simulink model "Sensors"  (Simulink 8.8)
settings: Solver=ode45  StartTime=0.0  StopTime=10.0  RelTol=1e-3  EnableMultiTasking=on
undefined symbols (not defined in the file): Amc_flgAirMassFlowOverride, Amc_uSensMaxValid, Amc_uSensMinValid, Bvc_rVoltDivHigh, Bvc_rVoltDivLow, Bvc_uBattMax, Bvc_uBattMin, Cpc_flgPChargeOverride, Ctc_rPullUp_C, Ctc_uSensMaxValid, Ctc_uSensMinValid, Ctc_uSupply, Egc_facEgasMan, Egc_flgEgasOverride, Egc_stEgasFilt, Egc_tiTEgasFilt, Egc_uSensMaxValid, Egc_uSensMinValid, Mpc_uSensMaxValid, Mpc_uSensMinValid, Mtc_rPullUp_C, Mtc_uSensMaxValid, Mtc_uSensMinValid, Mtc_uSupply, Opc_rpmEngMinOilPressure
libraries: simulink x8
(part 1 of 2)
settings Model: Creator=YAL9FE  LastModifiedBy=ADM4KOR
settings OptimizationCC: ExpressionDepthLimit=2147483647
settings DebuggingCC: SolverPrmCheckMsg=warning
settings ConfigComp: CovSFcnEnable=off

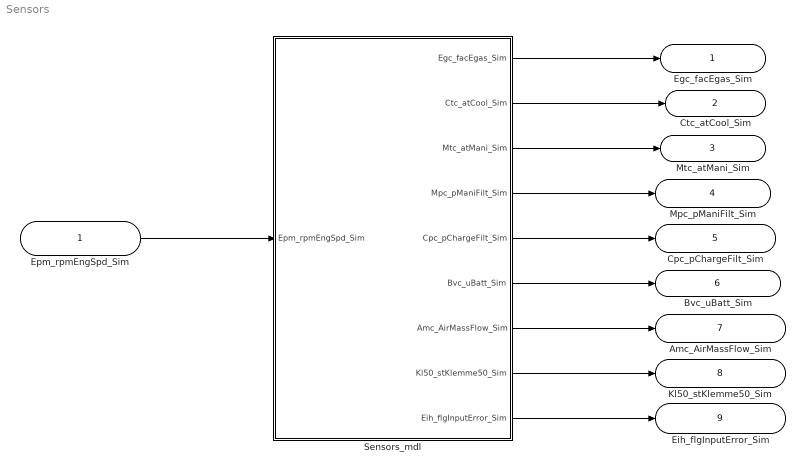
== system Sensors ==
  Epm_rpmEngSpd_Sim : Inport
  Sensors_mdl : Subsystem
  Egc_facEgas_Sim : Outport
  Ctc_atCool_Sim : Outport  Port=2
  Mtc_atMani_Sim : Outport  Port=3
  Mpc_pManiFilt_Sim : Outport  Port=4
  Cpc_pChargeFilt_Sim : Outport  Port=5
  Bvc_uBatt_Sim : Outport  Port=6
  Amc_AirMassFlow_Sim : Outport  Port=7
  Kl50_stKlemme50_Sim : Outport  Port=8
  Eih_flgInputError_Sim : Outport  Port=9
  wires:
  Epm_rpmEngSpd_Sim/1 -> Sensors_mdl/1(Epm_rpmEngSpd_Sim)
  Sensors_mdl/1(Egc_facEgas_Sim) -> Egc_facEgas_Sim/1
  Sensors_mdl/2(Ctc_atCool_Sim) -> Ctc_atCool_Sim/1
  Sensors_mdl/3(Mtc_atMani_Sim) -> Mtc_atMani_Sim/1
  Sensors_mdl/4(Mpc_pManiFilt_Sim) -> Mpc_pManiFilt_Sim/1
  Sensors_mdl/5(Cpc_pChargeFilt_Sim) -> Cpc_pChargeFilt_Sim/1
  Sensors_mdl/6(Bvc_uBatt_Sim) -> Bvc_uBatt_Sim/1
  Sensors_mdl/7(Amc_AirMassFlow_Sim) -> Amc_AirMassFlow_Sim/1
  Sensors_mdl/8(Kl50_stKlemme50_Sim) -> Kl50_stKlemme50_Sim/1
  Sensors_mdl/9(Eih_flgInputError_Sim) -> Eih_flgInputError_Sim/1

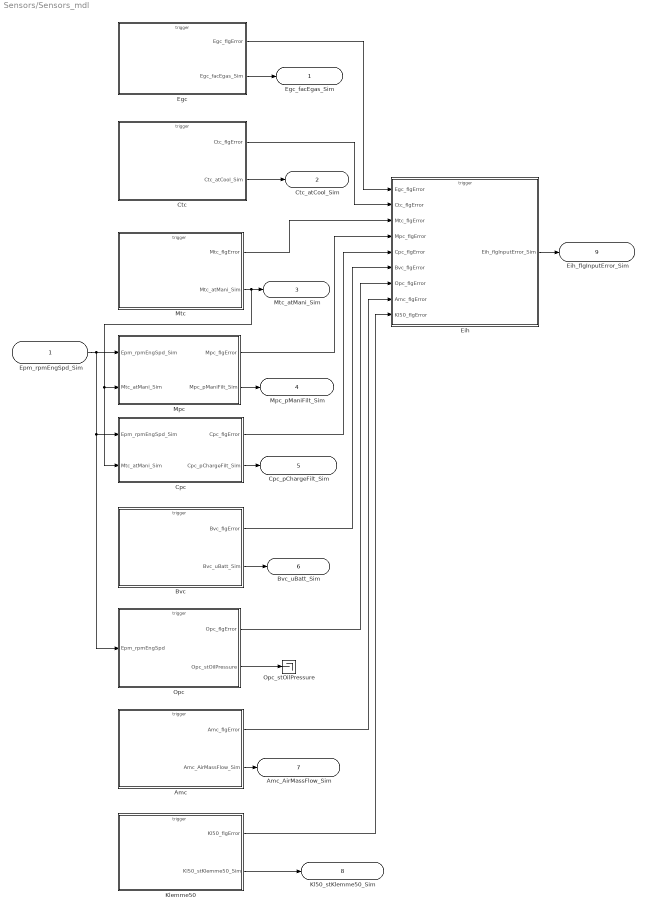
== system Sensors/Sensors_mdl ==
  Epm_rpmEngSpd_Sim : Inport
  Amc : Subsystem  mask(Sensors){}
      mask help: AirMassFlowMeter
      mask Display:
      | image(imread('AirMassFlowMeter.jpg'))
      | port_label('output',1,'Amc_flgError')
      | port_label('output',2,'Amc_AirMassFlow_Sim')
  Bvc : Subsystem  mask(Sensors){}
      mask help: BatteryVoltage
      mask Display:
      | image(imread('BatteryVoltage.jpg'))
      | port_label('output',1,'Bvc_flgError')
      | port_label('output',2,'Bvc_uBatt_Sim')
  Cpc : Subsystem  mask(Sensors){}
      mask help: ChargingPressure
      mask Display:
      | image(imread('ChargingPressure.jpg'))
      | port_label('input',1,'Epm_rpmEngSpd_Sim')
      | port_label('input',2,'Mtc_atMani_Sim')
      | port_label('output',1,'Cpc_flgError')
      | port_label('output',2,'Cpc_pChargeFilt_Sim')
  Ctc : Subsystem  mask(Sensors){}
      mask help: CoolantTemperature
      mask Display:
      | image(imread('CoolantTemperature.jpg'))
      | port_label('output',1,'Ctc_flgError')
      | port_label('output',2,'Ctc_atCool_Sim')
  Egc : Subsystem  mask(Sensors){}
      mask help: Egas
      mask Display:
      | image(imread('Egas.jpg'))
      | port_label('output',1,'Egc_flgError')
      | port_label('output',2,'Egc_facEgas_Sim')
  Eih : Subsystem  mask(Functions){}
      mask help: ErrorInput
      mask Display:
      | image(imread('ErrorInput.jpg'))
      | port_label('input',1,'Egc_flgError')
      | port_label('input',2,'Ctc_flgError')
      | port_label('input',3,'Mtc_flgError')
      | port_label('input',4,'Mpc_flgError')
      | port_label('input',5,'Cpc_flgError')
      | port_label('input',6,'Bvc_flgError')
      | port_label('input',7,'Opc_flgError')
      | port_label('input',8,'Amc_flgError')
      | port_label('input',9,'Kl50_flgError')
      | port_label('output',1,'Eih_flgInputError_Sim')
  Klemme50 : Subsystem  mask(Sensors){}
      mask help: Klemme50
      mask Display:
      | image(imread('Klemme50.jpg'))
      | port_label('output',1,'Kl50_flgError')
      | port_label('output',2,'Kl50_stKlemme50_Sim')
  Mpc : Subsystem  mask(Sensors){}
      mask help: ManifoldPressure
      mask Display:
      | image(imread('ManifoldPressure.jpg'))
      | port_label('input',1,'Epm_rpmEngSpd_Sim')
      | port_label('input',2,'Mtc_atMani_Sim')
      | port_label('output',1,'Mpc_flgError')
      | port_label('output',2,'Mpc_pManiFilt_Sim')
  Mtc : Subsystem  mask(Sensors){}
      mask help: ManifoldTemperature
      mask Display:
      | image(imread('ManifoldTemperature.jpg'))
      | port_label('output',1,'Mtc_flgError')
      | port_label('output',2,'Mtc_atMani_Sim')
  Opc : Subsystem  mask(Sensors){}
      mask help: OilPressure
      mask Display:
      | image(imread('OilPressure.jpg'))
      | port_label('input',1,'Epm_rpmEngSpd')
      | port_label('output',1,'Opc_flgError')
      | port_label('output',2,'Opc_stOilPressure')
  Opc_stOilPressure : Terminator
  Egc_facEgas_Sim : Outport
  Ctc_atCool_Sim : Outport  Port=2
  Mtc_atMani_Sim : Outport  Port=3
  Mpc_pManiFilt_Sim : Outport  Port=4
  Cpc_pChargeFilt_Sim : Outport  Port=5
  Bvc_uBatt_Sim : Outport  Port=6
  Amc_AirMassFlow_Sim : Outport  Port=7
  Kl50_stKlemme50_Sim : Outport  Port=8
  Eih_flgInputError_Sim : Outport  Port=9
  wires:
  Eih/1(Eih_flgInputError_Sim) -> Eih_flgInputError_Sim/1
  Egc/2(Egc_facEgas_Sim) -> Egc_facEgas_Sim/1
  Egc/1(Egc_flgError) -> Eih/1(Egc_flgError)
  Cpc/1(Cpc_flgError) -> Eih/5(Cpc_flgError)
  Mpc/2(Mpc_pManiFilt_Sim) -> Mpc_pManiFilt_Sim/1
  Klemme50/2(Kl50_stKlemme50_Sim) -> Kl50_stKlemme50_Sim/1
  Ctc/1(Ctc_flgError) -> Eih/2(Ctc_flgError)
  Ctc/2(Ctc_atCool_Sim) -> Ctc_atCool_Sim/1
  Mtc/1(Mtc_flgError) -> Eih/3(Mtc_flgError)
  Mtc/2(Mtc_atMani_Sim) -> Mtc_atMani_Sim/1, Cpc/2(Mtc_atMani_Sim), Mpc/2(Mtc_atMani_Sim)
  Mpc/1(Mpc_flgError) -> Eih/4(Mpc_flgError)
  Klemme50/1(Kl50_flgError) -> Eih/9(Kl50_flgError)
  Amc/2(Amc_AirMassFlow_Sim) -> Amc_AirMassFlow_Sim/1
  Epm_rpmEngSpd_Sim/1 -> Opc/1(Epm_rpmEngSpd), Cpc/1(Epm_rpmEngSpd_Sim), Mpc/1(Epm_rpmEngSpd_Sim)
  Bvc/1(Bvc_flgError) -> Eih/6(Bvc_flgError)
  Bvc/2(Bvc_uBatt_Sim) -> Bvc_uBatt_Sim/1
  Opc/1(Opc_flgError) -> Eih/7(Opc_flgError)
  Opc/2(Opc_stOilPressure) -> Opc_stOilPressure/1
  Cpc/2(Cpc_pChargeFilt_Sim) -> Cpc_pChargeFilt_Sim/1
  Amc/1(Amc_flgError) -> Eih/8(Amc_flgError)

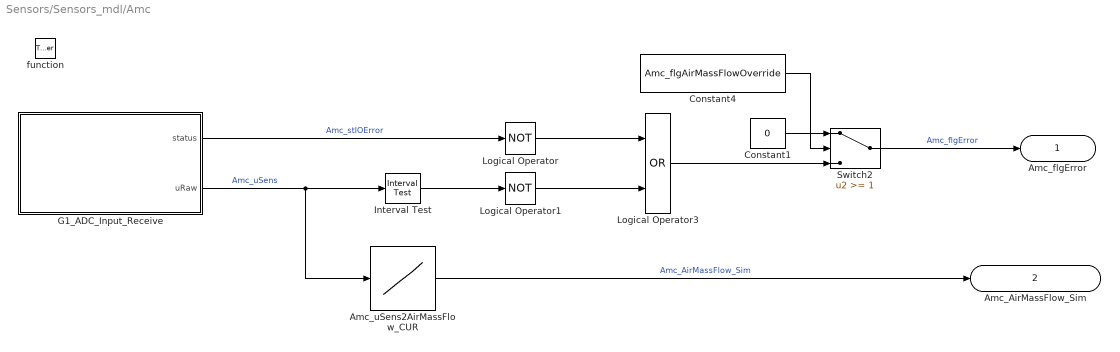
== system Sensors/Sensors_mdl/Amc ==
  function : TriggerPort  TriggerType=function-call  VariantControl=(inherit)
  Amc_uSens2AirMassFlow_CUR : Lookup_n-D  NumberOfTableDimensions=1  BreakpointsForDimension1=[1:3]  BreakpointsForDimension1DataTypeStr=Inherit: Inherit from 'Breakpoint data'  Table=[1 3 7]  TableDataTypeStr=Inherit: Inherit from 'Table data'  ExtrapMethod=Clip  OutDataTypeStr=Inherit: Inherit from 'Table data'  InputSameDT=on
  Constant1 : Constant  Value=0  OutDataTypeStr=boolean
  Constant4 : Constant  Value=Amc_flgAirMassFlowOverride
  G1_ADC_Input_Receive : Subsystem  mask{ChannelName=I_A_AN21}
      mask prompts: ChannelName "Channel name"
      mask init:
      | ehooks_medc17flex_devlib_io_block('mask_init');
      settings: AttributesFormatString=Channel name: '%<ChannelName>'
      mask TypeOptions ChannelName: <empty> | I_A_AN01 | I_A_AN02 | I_A_AN03 | I_A_AN05 | I_A_AN06 | I_A_AN07 | I_A_AN08 | I_A_AN10 | I_A_AN11 | I_A_AN12 | I_A_AN13 | I_A_AN14 | I_A_AN15 | I_A_AN16 | I_A_AN17 | I_A_AN18 | I_A_AN19 | I_A_AN20 | I_A_AN21 | I_A_AN23 | I_A_AN32 | I_A_AN35 | I_A_AN36 | I_A_AN37 | I_A_AN39 | I_A_AN100 | I_A_AN101 | I_A_AN103 | I_A_AN104 | I_A_AN105 | I_A_AN106
      mask Display: image(imread('Input_Analog.jpg'))
  Interval Test : simulink/Logic and Bit Operations/Interval Test  IntervalClosedRight=on  uplimit=Amc_uSensMaxValid  IntervalClosedLeft=on  lowlimit=Amc_uSensMinValid  OutDataTypeStr=boolean
  Logical Operator : Logic  Operator=NOT  AllPortsSameDT=off  OutDataTypeStr=boolean
  Logical Operator1 : Logic  Operator=NOT  AllPortsSameDT=off  OutDataTypeStr=boolean
  Logical Operator3 : Logic  Operator=OR  AllPortsSameDT=off  OutDataTypeStr=boolean
  Switch2 : Switch  Threshold=1
  Amc_flgError : Outport
  Amc_AirMassFlow_Sim : Outport  Port=2
  wires:
  G1_ADC_Input_Receive/1(status) -> Logical Operator/1  "Amc_stIOError"
  G1_ADC_Input_Receive/2(uRaw) -> Amc_uSens2AirMassFlow_CUR/1, Interval Test/1  "Amc_uSens"
  Interval Test/1 -> Logical Operator1/1
  Logical Operator/1 -> Logical Operator3/1
  Logical Operator1/1 -> Logical Operator3/2
  Switch2/1 -> Amc_flgError/1  "Amc_flgError"
  Amc_uSens2AirMassFlow_CUR/1 -> Amc_AirMassFlow_Sim/1  "Amc_AirMassFlow_Sim"
  Constant1/1 -> Switch2/1
  Logical Operator3/1 -> Switch2/3
  Constant4/1 -> Switch2/2

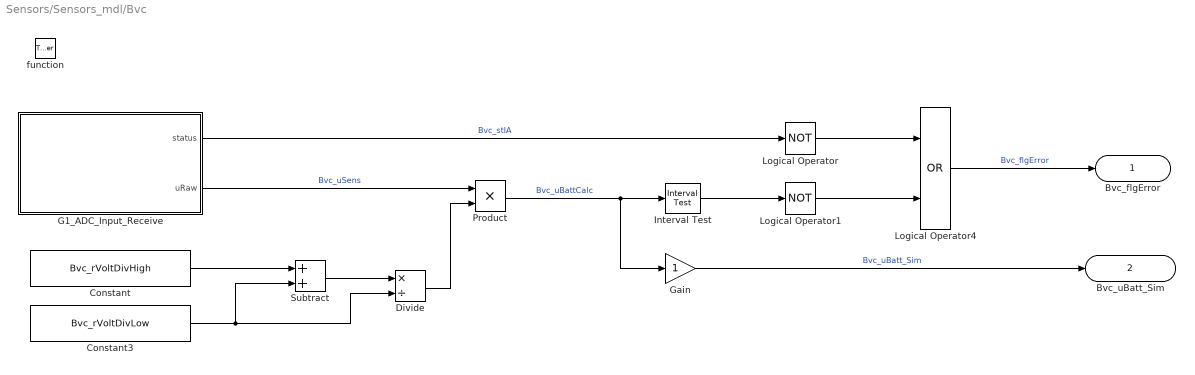
== system Sensors/Sensors_mdl/Bvc ==
  function : TriggerPort  TriggerType=function-call  VariantControl=(inherit)
  Constant : Constant  Value=Bvc_rVoltDivHigh
  Constant3 : Constant  Value=Bvc_rVoltDivLow
  Divide : Product  Inputs=*/  OutDataTypeStr=Inherit: Same as first input
  G1_ADC_Input_Receive : Subsystem  mask{ChannelName=I_A_AN16}
      mask prompts: ChannelName "Channel name"
      mask init:
      | ehooks_medc17flex_devlib_io_block('mask_init');
      settings: AttributesFormatString=Channel name: '%<ChannelName>'
      mask TypeOptions ChannelName: <empty> | I_A_AN01 | I_A_AN02 | I_A_AN03 | I_A_AN05 | I_A_AN06 | I_A_AN07 | I_A_AN08 | I_A_AN10 | I_A_AN11 | I_A_AN12 | I_A_AN13 | I_A_AN14 | I_A_AN15 | I_A_AN16 | I_A_AN17 | I_A_AN18 | I_A_AN19 | I_A_AN20 | I_A_AN21 | I_A_AN23 | I_A_AN32 | I_A_AN35 | I_A_AN36 | I_A_AN37 | I_A_AN39 | I_A_AN100 | I_A_AN101 | I_A_AN103 | I_A_AN104 | I_A_AN105 | I_A_AN106
      mask Display: image(imread('Input_Analog.jpg'))
  Gain : Gain
  Interval Test : simulink/Logic and Bit Operations/Interval Test  IntervalClosedRight=on  uplimit=Bvc_uBattMax  IntervalClosedLeft=on  lowlimit=Bvc_uBattMin  OutDataTypeStr=boolean
  Logical Operator : Logic  Operator=NOT  AllPortsSameDT=off  OutDataTypeStr=boolean
  Logical Operator1 : Logic  Operator=NOT  AllPortsSameDT=off  OutDataTypeStr=boolean
  Logical Operator4 : Logic  Operator=OR  AllPortsSameDT=off  OutDataTypeStr=boolean
  Product : Product  OutDataTypeStr=Inherit: Same as first input
  Subtract : Sum  OutDataTypeStr=Inherit: Same as first input
  Bvc_flgError : Outport
  Bvc_uBatt_Sim : Outport  Port=2
  wires:
  G1_ADC_Input_Receive/1(status) -> Logical Operator/1  "Bvc_stIA"
  Interval Test/1 -> Logical Operator1/1
  Logical Operator/1 -> Logical Operator4/1
  Logical Operator1/1 -> Logical Operator4/2
  Logical Operator4/1 -> Bvc_flgError/1  "Bvc_flgError"
  Constant/1 -> Subtract/1
  Constant3/1 -> Subtract/2, Divide/2
  Subtract/1 -> Divide/1
  Product/1 -> Gain/1, Interval Test/1  "Bvc_uBattCalc"
  G1_ADC_Input_Receive/2(uRaw) -> Product/1  "Bvc_uSens"
  Divide/1 -> Product/2
  Gain/1 -> Bvc_uBatt_Sim/1  "Bvc_uBatt_Sim"

== system Sensors/Sensors_mdl/Cpc ==
  Epm_rpmEngSpd_Sim : Inport
  Mtc_atMani_Sim : Inport  Port=2
  Cpc_calc : Subsystem  mask(Sensors){}
      mask help: ChargingPressureCalc
      mask Display:
      | image(imread('ManifoldPressure.jpg'))
      | port_label('input',1,'Epm_rpmEngSpd')
      | port_label('input',2,'Cpc_pMani')
      | port_label('input',3,'Cpc_flgError')
      | port_label('output',1,'Cpc_pChargeFilt_Sim')
  Cpc_get : Subsystem  mask(Sensors){}
      mask help: ChargingPressureGet
      mask Display:
      | image(imread('ManifoldPressure.jpg'))
      | port_label('input',1,'Mtc_atMani')
      | port_label('output',1,'Cpc_flgError')
      | port_label('output',2,'Cpc_pMani')
  Cpc_flgError : Outport
  Cpc_pChargeFilt_Sim : Outport  Port=2
  wires:
  Cpc_calc/1(Cpc_pChargeFilt_Sim) -> Cpc_pChargeFilt_Sim/1
  Cpc_get/2(Cpc_pMani) -> Cpc_calc/2(Cpc_pMani)
  Epm_rpmEngSpd_Sim/1 -> Cpc_calc/1(Epm_rpmEngSpd_Sim)
  Cpc_get/1(Cpc_flgError) -> Cpc_calc/3(Cpc_flgError), Cpc_flgError/1
  Mtc_atMani_Sim/1 -> Cpc_get/1(Mtc_atMani_Sim)

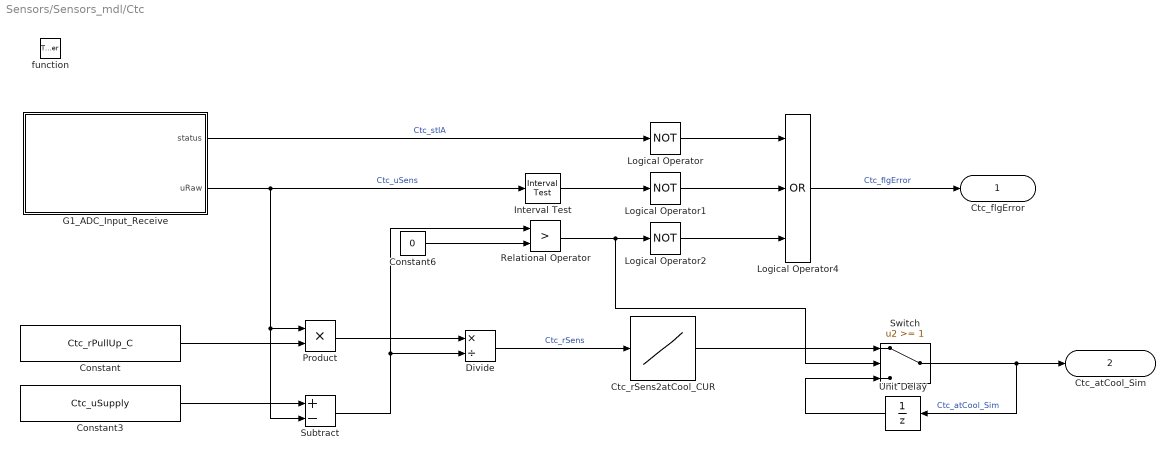
== system Sensors/Sensors_mdl/Ctc ==
  function : TriggerPort  TriggerType=function-call  VariantControl=(inherit)
  Constant : Constant  Value=Ctc_rPullUp_C
  Constant3 : Constant  Value=Ctc_uSupply
  Constant6 : Constant  Value=0  OutDataTypeStr=single
  Ctc_rSens2atCool_CUR : Lookup_n-D  NumberOfTableDimensions=1  BreakpointsForDimension1=[1:3]  BreakpointsForDimension1DataTypeStr=Inherit: Inherit from 'Breakpoint data'  Table=[1 3 4 ]  TableDataTypeStr=Inherit: Inherit from 'Table data'  ExtrapMethod=Clip  OutDataTypeStr=Inherit: Inherit from 'Table data'  InputSameDT=on
  Divide : Product  Inputs=*/  OutDataTypeStr=Inherit: Same as first input
  G1_ADC_Input_Receive : Subsystem  mask{ChannelName=I_A_AN10}
      mask prompts: ChannelName "Channel name"
      mask init:
      | ehooks_medc17flex_devlib_io_block('mask_init');
      settings: AttributesFormatString=Channel name: '%<ChannelName>'
      mask TypeOptions ChannelName: <empty> | I_A_AN01 | I_A_AN02 | I_A_AN03 | I_A_AN05 | I_A_AN06 | I_A_AN07 | I_A_AN08 | I_A_AN10 | I_A_AN11 | I_A_AN12 | I_A_AN13 | I_A_AN14 | I_A_AN15 | I_A_AN16 | I_A_AN17 | I_A_AN18 | I_A_AN19 | I_A_AN20 | I_A_AN21 | I_A_AN23 | I_A_AN32 | I_A_AN35 | I_A_AN36 | I_A_AN37 | I_A_AN39 | I_A_AN100 | I_A_AN101 | I_A_AN103 | I_A_AN104 | I_A_AN105 | I_A_AN106
      mask Display: image(imread('Input_Analog.jpg'))
  Interval Test : simulink/Logic and Bit Operations/Interval Test  IntervalClosedRight=on  uplimit=Ctc_uSensMaxValid  IntervalClosedLeft=on  lowlimit=Ctc_uSensMinValid  OutDataTypeStr=boolean
  Logical Operator : Logic  Operator=NOT  AllPortsSameDT=off  OutDataTypeStr=boolean
  Logical Operator1 : Logic  Operator=NOT  AllPortsSameDT=off  OutDataTypeStr=boolean
  Logical Operator2 : Logic  Operator=NOT  AllPortsSameDT=off  OutDataTypeStr=boolean
  Logical Operator4 : Logic  Operator=OR  Inputs=3  AllPortsSameDT=off  OutDataTypeStr=boolean
  Product : Product  OutDataTypeStr=Inherit: Same as first input
  Relational Operator : RelationalOperator  Operator=>  OutDataTypeStr=boolean  RndMeth=Nearest
  Subtract : Sum  Inputs=+-  OutDataTypeStr=Inherit: Same as first input
  Switch : Switch  Threshold=1
  Unit Delay : UnitDelay  SampleTime=-1
  Ctc_flgError : Outport
  Ctc_atCool_Sim : Outport  Port=2
  wires:
  Logical Operator4/1 -> Ctc_flgError/1  "Ctc_flgError"
  Logical Operator1/1 -> Logical Operator4/2
  Logical Operator/1 -> Logical Operator4/1
  Interval Test/1 -> Logical Operator1/1
  G1_ADC_Input_Receive/2(uRaw) -> Subtract/2, Product/1, Interval Test/1  "Ctc_uSens"
  G1_ADC_Input_Receive/1(status) -> Logical Operator/1  "Ctc_stIA"
  Constant/1 -> Product/2
  Constant3/1 -> Subtract/1
  Product/1 -> Divide/1
  Subtract/1 -> Divide/2, Relational Operator/1
  Constant6/1 -> Relational Operator/2
  Relational Operator/1 -> Logical Operator2/1, Switch/2
  Logical Operator2/1 -> Logical Operator4/3
  Switch/1 -> Ctc_atCool_Sim/1, Unit Delay/1  "Ctc_atCool_Sim"
  Unit Delay/1 -> Switch/3
  Ctc_rSens2atCool_CUR/1 -> Switch/1
  Divide/1 -> Ctc_rSens2atCool_CUR/1  "Ctc_rSens"

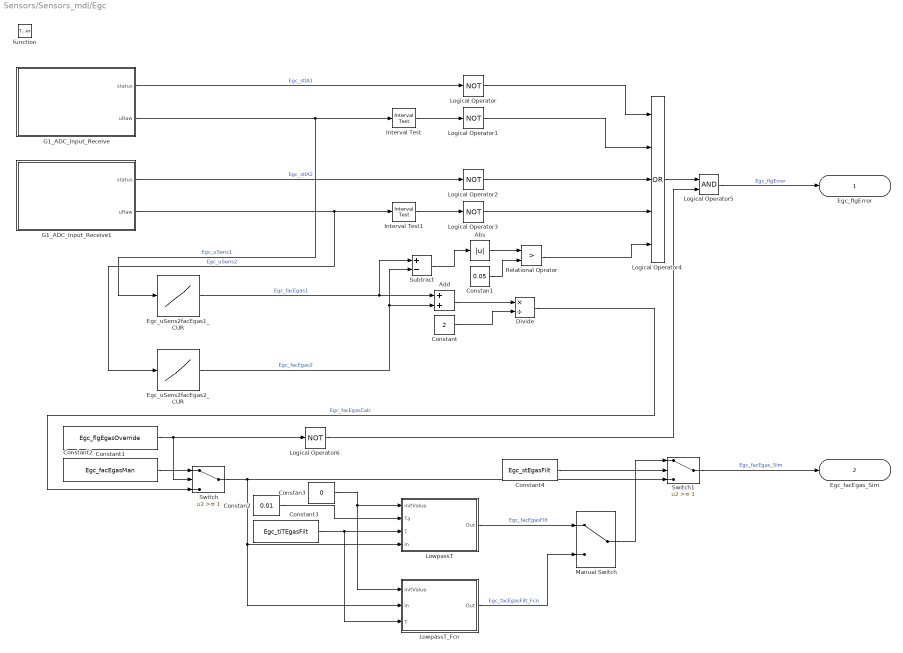
== system Sensors/Sensors_mdl/Egc ==
  function : TriggerPort  TriggerType=function-call  VariantControl=(inherit)
  Abs : Abs
  Add : Sum  OutDataTypeStr=Inherit: Same as first input
  Constan1 : Constant  Value=0.05  OutDataTypeStr=single
  Constan2 : Constant  Value=0.01  OutMin=0  OutDataTypeStr=single
  Constan3 : Constant  Value=0  OutDataTypeStr=single
  Constant : Constant  Value=2  OutDataTypeStr=single
  Constant1 : Constant  Value=Egc_flgEgasOverride
  Constant2 : Constant  Value=Egc_facEgasMan
  Constant3 : Constant  Value=Egc_tiTEgasFilt
  Constant4 : Constant  Value=Egc_stEgasFilt
  Divide : Product  Inputs=*/  OutDataTypeStr=Inherit: Same as first input
  Egc_uSens2facEgas1_CUR : Lookup_n-D  NumberOfTableDimensions=1  BreakpointsForDimension1=[1:3]  BreakpointsForDimension1DataTypeStr=Inherit: Inherit from 'Breakpoint data'  Table=[1 3 9]  TableDataTypeStr=Inherit: Inherit from 'Table data'  ExtrapMethod=Clip  OutDataTypeStr=Inherit: Inherit from 'Table data'  InputSameDT=on
  Egc_uSens2facEgas2_CUR : Lookup_n-D  NumberOfTableDimensions=1  BreakpointsForDimension1=[1:4]  BreakpointsForDimension1DataTypeStr=Inherit: Inherit from 'Breakpoint data'  Table=[1 3 7 9]  TableDataTypeStr=Inherit: Inherit from 'Table data'  ExtrapMethod=Clip  OutDataTypeStr=Inherit: Inherit from 'Table data'  InputSameDT=on
  G1_ADC_Input_Receive : Subsystem  mask{ChannelName=I_A_AN08}
      mask prompts: ChannelName "Channel name"
      mask init:
      | ehooks_medc17flex_devlib_io_block('mask_init');
      settings: AttributesFormatString=Channel name: '%<ChannelName>'
      mask TypeOptions ChannelName: <empty> | I_A_AN01 | I_A_AN02 | I_A_AN03 | I_A_AN05 | I_A_AN06 | I_A_AN07 | I_A_AN08 | I_A_AN10 | I_A_AN11 | I_A_AN12 | I_A_AN13 | I_A_AN14 | I_A_AN15 | I_A_AN16 | I_A_AN17 | I_A_AN18 | I_A_AN19 | I_A_AN20 | I_A_AN21 | I_A_AN23 | I_A_AN32 | I_A_AN35 | I_A_AN36 | I_A_AN37 | I_A_AN39 | I_A_AN100 | I_A_AN101 | I_A_AN103 | I_A_AN104 | I_A_AN105 | I_A_AN106
      mask Display: image(imread('Input_Analog.jpg'))
  G1_ADC_Input_Receive1 : Subsystem  mask{ChannelName=I_A_AN13}
      mask prompts: ChannelName "Channel name"
      mask init:
      | ehooks_medc17flex_devlib_io_block('mask_init');
      settings: AttributesFormatString=Channel name: '%<ChannelName>'
      mask TypeOptions ChannelName: <empty> | I_A_AN01 | I_A_AN02 | I_A_AN03 | I_A_AN05 | I_A_AN06 | I_A_AN07 | I_A_AN08 | I_A_AN10 | I_A_AN11 | I_A_AN12 | I_A_AN13 | I_A_AN14 | I_A_AN15 | I_A_AN16 | I_A_AN17 | I_A_AN18 | I_A_AN19 | I_A_AN20 | I_A_AN21 | I_A_AN23 | I_A_AN32 | I_A_AN35 | I_A_AN36 | I_A_AN37 | I_A_AN39 | I_A_AN100 | I_A_AN101 | I_A_AN103 | I_A_AN104 | I_A_AN105 | I_A_AN106
      mask Display: image(imread('Input_Analog.jpg'))
  Interval Test : simulink/Logic and Bit Operations/Interval Test  IntervalClosedRight=on  uplimit=Egc_uSensMaxValid  IntervalClosedLeft=on  lowlimit=Egc_uSensMinValid  OutDataTypeStr=boolean
  Interval Test1 : simulink/Logic and Bit Operations/Interval Test  IntervalClosedRight=on  uplimit=Egc_uSensMaxValid  IntervalClosedLeft=on  lowlimit=Egc_uSensMinValid  OutDataTypeStr=boolean
  Logical Operator{,1..3,6} (5 alike) : Logic  Operator=NOT  AllPortsSameDT=off  OutDataTypeStr=boolean
  Logical Operator4 : Logic  Operator=OR  Inputs=5  AllPortsSameDT=off  OutDataTypeStr=boolean
  Logical Operator5 : Logic  AllPortsSameDT=off  OutDataTypeStr=boolean
  LowpassT : Subsystem
      mask help: LowpassT
      mask Display: image(imread('LowpassT.jpg'))
  LowpassT_Fcn : Subsystem
      mask help: LowpassT_Fcn
      mask Display: image(imread('LowpassT.jpg'))
  Manual Switch : ManualSwitch
  Relational Oprator : RelationalOperator  Operator=>  OutDataTypeStr=boolean  RndMeth=Nearest
  Subtract : Sum  Inputs=+-  OutDataTypeStr=Inherit: Same as first input
  Switch : Switch  Threshold=1
  Switch1 : Switch  Threshold=1
  Egc_flgError : Outport  InitialOutput=0.0
  Egc_facEgas_Sim : Outport  Port=2  InitialOutput=0.0
  wires:
  Manual Switch/1 -> Switch1/1
  LowpassT/1(Out) -> Manual Switch/1  "Egc_facEgasFilt"
  LowpassT_Fcn/1(Out) -> Manual Switch/2  "Egc_facEgasFilt_Fcn"
  Constant3/1 -> LowpassT_Fcn/3(T), LowpassT/3(T)
  Constan2/1 -> LowpassT/2(Ta)
  Constan3/1 -> LowpassT_Fcn/1(initValue), LowpassT/1(initValue)
  G1_ADC_Input_Receive1/2(uRaw) -> Egc_uSens2facEgas2_CUR/1, Interval Test1/1  "Egc_uSens2"
  G1_ADC_Input_Receive/2(uRaw) -> Egc_uSens2facEgas1_CUR/1, Interval Test/1  "Egc_uSens1"
  Divide/1 -> Switch/3  "Egc_facEgasCalc"
  G1_ADC_Input_Receive/1(status) -> Logical Operator/1  "Egc_stIA1"
  Interval Test/1 -> Logical Operator1/1
  Interval Test1/1 -> Logical Operator3/1
  Logical Operator/1 -> Logical Operator4/1
  Logical Operator1/1 -> Logical Operator4/2
  Logical Operator2/1 -> Logical Operator4/3
  Logical Operator3/1 -> Logical Operator4/4
  Logical Operator4/1 -> Logical Operator5/1
  Logical Operator5/1 -> Egc_flgError/1  "Egc_flgError"
  Egc_uSens2facEgas1_CUR/1 -> Subtract/1, Add/1  "Egc_facEgas1"
  Egc_uSens2facEgas2_CUR/1 -> Subtract/2, Add/2  "Egc_facEgas2"
  Add/1 -> Divide/1
  Constant/1 -> Divide/2
  Subtract/1 -> Abs/1
  Abs/1 -> Relational Oprator/1
  Constan1/1 -> Relational Oprator/2
  Relational Oprator/1 -> Logical Operator4/5
  Constant1/1 -> Logical Operator6/1, Switch/2
  Logical Operator6/1 -> Logical Operator5/2
  Switch/1 -> Switch1/3, LowpassT_Fcn/2(In), LowpassT/4(in)
  Switch1/1 -> Egc_facEgas_Sim/1  "Egc_facEgas_Sim"
  Constant4/1 -> Switch1/2
  G1_ADC_Input_Receive1/1(status) -> Logical Operator2/1  "Egc_stIA2"
  Constant2/1 -> Switch/1

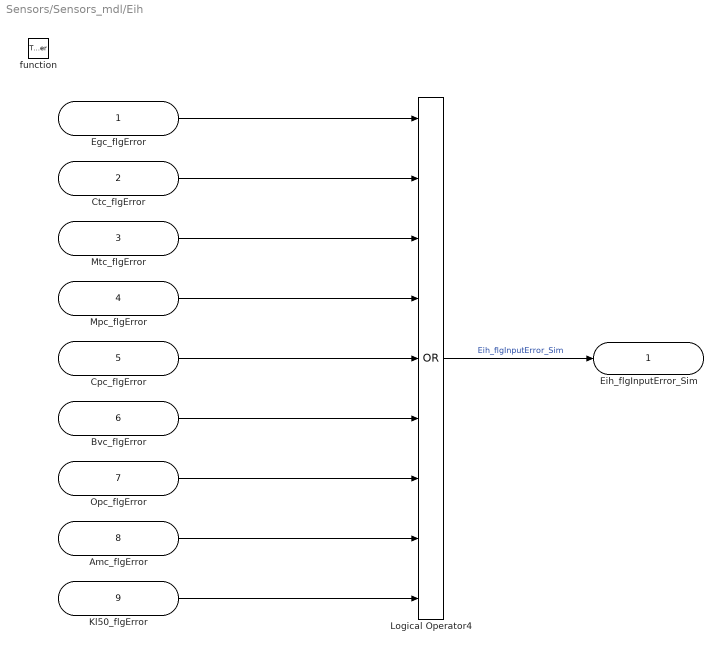
== system Sensors/Sensors_mdl/Eih ==
  Egc_flgError : Inport
  Ctc_flgError : Inport  Port=2
  Mtc_flgError : Inport  Port=3
  Mpc_flgError : Inport  Port=4
  Cpc_flgError : Inport  Port=5
  Bvc_flgError : Inport  Port=6
  Opc_flgError : Inport  Port=7
  Amc_flgError : Inport  Port=8
  Kl50_flgError : Inport  Port=9
  function : TriggerPort  TriggerType=function-call  VariantControl=(inherit)
  Logical Operator4 : Logic  Operator=OR  Inputs=9  AllPortsSameDT=off  OutDataTypeStr=boolean
  Eih_flgInputError_Sim : Outport
  wires:
  Logical Operator4/1 -> Eih_flgInputError_Sim/1  "Eih_flgInputError_Sim"
  Egc_flgError/1 -> Logical Operator4/1
  Ctc_flgError/1 -> Logical Operator4/2
  Mtc_flgError/1 -> Logical Operator4/3
  Mpc_flgError/1 -> Logical Operator4/4
  Cpc_flgError/1 -> Logical Operator4/5
  Bvc_flgError/1 -> Logical Operator4/6
  Opc_flgError/1 -> Logical Operator4/7
  Amc_flgError/1 -> Logical Operator4/8
  Kl50_flgError/1 -> Logical Operator4/9

== system Sensors/Sensors_mdl/Klemme50 ==
  function : TriggerPort  TriggerType=function-call  VariantControl=(inherit)
  G1_Digital_Input_Receive : Subsystem  AncestorBlock=ehooks_medc17flex_G1_lib/Library Blocks/Basic_IO/Inputs/G1_Digital_Input_Receive  mask{ChannelName=I_S_DIG17}
      mask prompts: ChannelName "Channel name"
      mask init:
      | ehooks_medc17flex_devlib_io_block('mask_init');
      settings: AttributesFormatString=Channel name: '%<ChannelName>'
      mask TypeOptions ChannelName: <empty> | I_S_T15 | I_S_DIG02 | I_S_DIG05 | I_S_DIG13 | I_S_DIG14 | I_S_DIG15 | I_S_DIG16 | I_S_DIG17 | I_S_DIG20 | I_S_DIG50
      mask Display: image(imread('Input_Digital.jpg'))
  Logical Operator : Logic  Operator=NOT  AllPortsSameDT=off  OutDataTypeStr=boolean
  Kl50_flgError : Outport
  Kl50_stKlemme50_Sim : Outport  Port=2
  wires:
  Logical Operator/1 -> Kl50_flgError/1  "Kl50_flgError"
  G1_Digital_Input_Receive/1(status) -> Logical Operator/1  "Kl50_stIO"
  G1_Digital_Input_Receive/2(stRaw1) -> Kl50_stKlemme50_Sim/1  "Kl50_stKlemme50_Sim"

== system Sensors/Sensors_mdl/Mpc ==
  Epm_rpmEngSpd_Sim : Inport
  Mtc_atMani_Sim : Inport  Port=2
  Mpc_calc : Subsystem  mask(Sensors){}
      mask help: ManifoldPressureCalc
      mask Display:
      | image(imread('ManifoldPressure.jpg'))
      | port_label('input',1,'Epm_rpmEngSpd')
      | port_label('input',2,'Mpc_pMani')
      | port_label('input',3,'Mpc_flgError')
      | port_label('output',1,'Mpc_pManiFilt')
  Mpc_get : Subsystem  mask(Sensors){}
      mask help: ManifoldPressureGet
      mask Display:
      | image(imread('ManifoldPressure.jpg'))
      | port_label('input',1,'Mtc_atMani_Sim')
      | port_label('output',1,'Mpc_flgError')
      | port_label('output',2,'Mpc_pMani')
  Mpc_flgError : Outport
  Mpc_pManiFilt_Sim : Outport  Port=2
  wires:
  Mtc_atMani_Sim/1 -> Mpc_get/1(Mtc_atMani_Sim)
  Mpc_get/1(Mpc_flgError) -> Mpc_flgError/1, Mpc_calc/3(Mpc_flgError)
  Epm_rpmEngSpd_Sim/1 -> Mpc_calc/1(Epm_rpmEngSpd_Sim)
  Mpc_get/2(Mpc_pMani) -> Mpc_calc/2(Mpc_pMani)
  Mpc_calc/1(Mpc_pManiFilt_Sim) -> Mpc_pManiFilt_Sim/1

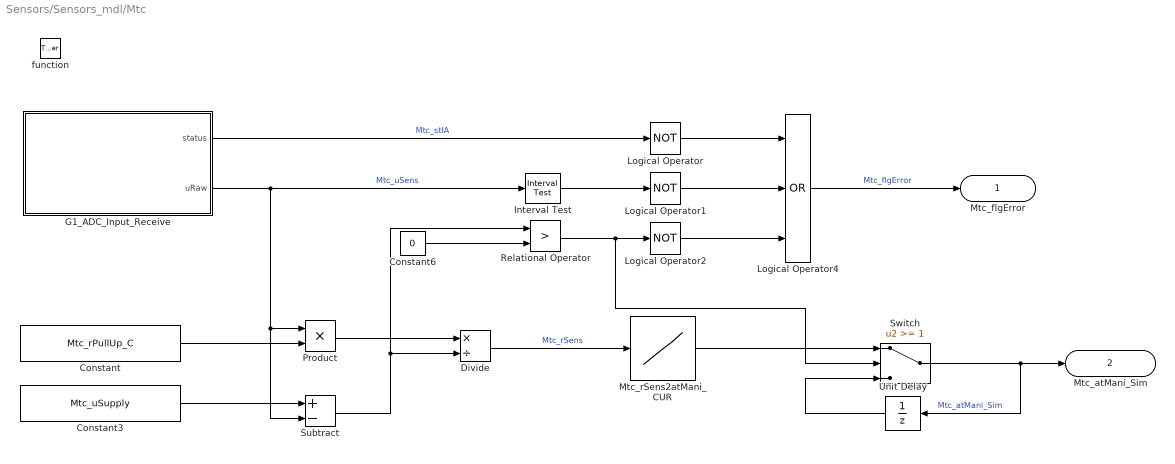
== system Sensors/Sensors_mdl/Mtc ==
  function : TriggerPort  TriggerType=function-call  VariantControl=(inherit)
  Constant : Constant  Value=Mtc_rPullUp_C
  Constant3 : Constant  Value=Mtc_uSupply
  Constant6 : Constant  Value=0  OutDataTypeStr=single
  Divide : Product  Inputs=*/  OutDataTypeStr=single
  G1_ADC_Input_Receive : Subsystem  mask{ChannelName=I_A_AN14}
      mask prompts: ChannelName "Channel name"
      mask init:
      | ehooks_medc17flex_devlib_io_block('mask_init');
      settings: AttributesFormatString=Channel name: '%<ChannelName>'
      mask TypeOptions ChannelName: <empty> | I_A_AN01 | I_A_AN02 | I_A_AN03 | I_A_AN05 | I_A_AN06 | I_A_AN07 | I_A_AN08 | I_A_AN10 | I_A_AN11 | I_A_AN12 | I_A_AN13 | I_A_AN14 | I_A_AN15 | I_A_AN16 | I_A_AN17 | I_A_AN18 | I_A_AN19 | I_A_AN20 | I_A_AN21 | I_A_AN23 | I_A_AN32 | I_A_AN35 | I_A_AN36 | I_A_AN37 | I_A_AN39 | I_A_AN100 | I_A_AN101 | I_A_AN103 | I_A_AN104 | I_A_AN105 | I_A_AN106
      mask Display: image(imread('Input_Analog.jpg'))
  Interval Test : simulink/Logic and Bit Operations/Interval Test  IntervalClosedRight=on  uplimit=Mtc_uSensMaxValid  IntervalClosedLeft=on  lowlimit=Mtc_uSensMinValid  OutDataTypeStr=boolean
  Logical Operator : Logic  Operator=NOT  AllPortsSameDT=off  OutDataTypeStr=boolean
  Logical Operator1 : Logic  Operator=NOT  AllPortsSameDT=off  OutDataTypeStr=boolean
  Logical Operator2 : Logic  Operator=NOT  AllPortsSameDT=off  OutDataTypeStr=boolean
  Logical Operator4 : Logic  Operator=OR  Inputs=3  AllPortsSameDT=off  OutDataTypeStr=boolean
  Mtc_rSens2atMani_CUR : Lookup_n-D  NumberOfTableDimensions=1  BreakpointsForDimension1=[1:3]  BreakpointsForDimension1DataTypeStr=Inherit: Inherit from 'Breakpoint data'  Table=[2 3 6]  TableDataTypeStr=Inherit: Inherit from 'Table data'  ExtrapMethod=Clip  OutDataTypeStr=Inherit: Inherit from 'Table data'  InputSameDT=on
  Product : Product  OutDataTypeStr=Inherit: Same as first input
  Relational Operator : RelationalOperator  Operator=>  OutDataTypeStr=boolean  RndMeth=Nearest
  Subtract : Sum  Inputs=+-  OutDataTypeStr=Inherit: Same as first input
  Switch : Switch  Threshold=1
  Unit Delay : UnitDelay  SampleTime=-1
  Mtc_flgError : Outport
  Mtc_atMani_Sim : Outport  Port=2
  wires:
  Mtc_rSens2atMani_CUR/1 -> Switch/1
  Unit Delay/1 -> Switch/3
  Switch/1 -> Unit Delay/1, Mtc_atMani_Sim/1  "Mtc_atMani_Sim"
  Logical Operator2/1 -> Logical Operator4/3
  Divide/1 -> Mtc_rSens2atMani_CUR/1  "Mtc_rSens"
  Relational Operator/1 -> Switch/2, Logical Operator2/1
  Constant6/1 -> Relational Operator/2
  Subtract/1 -> Relational Operator/1, Divide/2
  Product/1 -> Divide/1
  Constant3/1 -> Subtract/1
  Constant/1 -> Product/2
  G1_ADC_Input_Receive/1(status) -> Logical Operator/1  "Mtc_stIA"
  G1_ADC_Input_Receive/2(uRaw) -> Product/1, Subtract/2, Interval Test/1  "Mtc_uSens"
  Interval Test/1 -> Logical Operator1/1
  Logical Operator/1 -> Logical Operator4/1
  Logical Operator1/1 -> Logical Operator4/2
  Logical Operator4/1 -> Mtc_flgError/1  "Mtc_flgError"

== system Sensors/Sensors_mdl/Opc ==
  Epm_rpmEngSpd : Inport
  function : TriggerPort  TriggerType=function-call  VariantControl=(inherit)
  Constant : Constant  Value=Opc_rpmEngMinOilPressure
  G1_Digital_Input_Receive : Subsystem  AncestorBlock=ehooks_medc17flex_G1_lib/Library Blocks/Basic_IO/Inputs/G1_Digital_Input_Receive  mask{ChannelName=I_S_DIG13}
      mask prompts: ChannelName "Channel name"
      mask init:
      | ehooks_medc17flex_devlib_io_block('mask_init');
      settings: AttributesFormatString=Channel name: '%<ChannelName>'
      mask TypeOptions ChannelName: <empty> | I_S_T15 | I_S_DIG02 | I_S_DIG05 | I_S_DIG13 | I_S_DIG14 | I_S_DIG15 | I_S_DIG16 | I_S_DIG17 | I_S_DIG20 | I_S_DIG50
      mask Display: image(imread('Input_Digital.jpg'))
  Gain : Gain  OutDataTypeStr=Inherit: Same as input
  Logical Operator : Logic  Operator=NOT  AllPortsSameDT=off  OutDataTypeStr=boolean
  Logical Operator1 : Logic  Operator=NOT  AllPortsSameDT=off  OutDataTypeStr=boolean
  Logical Operator3 : Logic  AllPortsSameDT=off  OutDataTypeStr=boolean
  Logical Operator4 : Logic  Operator=OR  AllPortsSameDT=off  OutDataTypeStr=boolean
  Relational Operator : RelationalOperator  Operator=>  OutDataTypeStr=boolean  RndMeth=Nearest
  Opc_flgError : Outport
  Opc_stOilPressure : Outport  Port=2
  wires:
  Gain/1 -> Opc_stOilPressure/1  "Opc_stOilPressure"
  Constant/1 -> Relational Operator/2
  Logical Operator4/1 -> Opc_flgError/1  "Opc_flgError"
  Logical Operator/1 -> Logical Operator4/1
  G1_Digital_Input_Receive/1(status) -> Logical Operator/1  "Opc_stIA"
  Epm_rpmEngSpd/1 -> Relational Operator/1
  Relational Operator/1 -> Logical Operator3/1
  Logical Operator3/1 -> Logical Operator4/2
  Logical Operator1/1 -> Logical Operator3/2
  G1_Digital_Input_Receive/2(stRaw1) -> Logical Operator1/1, Gain/1  "Opc_stSens"

== system Sensors/Sensors_mdl/Amc/G1_ADC_Input_Receive ==
  Data Type Conversion2 : DataTypeConversion  OutMin=0.0  OutMax=5.0  OutDataTypeStr=single
  Data Type Conversion3 : DataTypeConversion  OutMin=0.0  OutMax=1.0  OutDataTypeStr=boolean
  FlexECU_DevLib_FcnAPI_Wrapper_SFcn : S-Function  FunctionName=ehooks_medc17flex_devlib_basic_io_fcncall  Parameters=NoInputPorts, NoOutputPorts, InputPortDataTypes, OutputPortDataTypes, CFunctionArgTypes, CFunctionName, ChannelName  SFunctionDeploymentMode=off  EnableBusSupport=off  mask{NoInputPorts=0, NoOutputPorts=2, InputPortDataTypes=, OutputPortDataTypes=uint8,int16, CFunctionArgTypes=ret,ref, CFunctionName=DevLib_Adc_Get, ChannelName=I_A_AN21}
      mask prompts: NoInputPorts "Number of input ports"; NoOutputPorts "Number of output ports"; InputPortDataTypes "Input port data types"; OutputPortDataTypes "Output port data types"; CFunctionArgTypes "C function argument types"; CFunctionName "C function name"; ChannelName "Channel (pin) name"
      mask Display: disp('EHOOKS FlexECU\nDevLib Wrapper\nS-Function')
  Gain : Gain  Gain=5/1023  OutDataTypeStr=Inherit: Same as input
  status : Outport
  uRaw : Outport  Port=2
  wires:
  Gain/1 -> uRaw/1
  Data Type Conversion2/1 -> Gain/1
  Data Type Conversion3/1 -> status/1
  FlexECU_DevLib_FcnAPI_Wrapper_SFcn/1 -> Data Type Conversion3/1
  FlexECU_DevLib_FcnAPI_Wrapper_SFcn/2 -> Data Type Conversion2/1

== system Sensors/Sensors_mdl/Bvc/G1_ADC_Input_Receive ==
  Data Type Conversion2 : DataTypeConversion  OutMin=0.0  OutMax=5.0  OutDataTypeStr=single
  Data Type Conversion3 : DataTypeConversion  OutMin=0.0  OutMax=1.0  OutDataTypeStr=boolean
  FlexECU_DevLib_FcnAPI_Wrapper_SFcn : S-Function  FunctionName=ehooks_medc17flex_devlib_basic_io_fcncall  Parameters=NoInputPorts, NoOutputPorts, InputPortDataTypes, OutputPortDataTypes, CFunctionArgTypes, CFunctionName, ChannelName  SFunctionDeploymentMode=off  EnableBusSupport=off  mask{NoInputPorts=0, NoOutputPorts=2, InputPortDataTypes=, OutputPortDataTypes=uint8,int16, CFunctionArgTypes=ret,ref, CFunctionName=DevLib_Adc_Get, ChannelName=I_A_AN16}
      mask prompts: NoInputPorts "Number of input ports"; NoOutputPorts "Number of output ports"; InputPortDataTypes "Input port data types"; OutputPortDataTypes "Output port data types"; CFunctionArgTypes "C function argument types"; CFunctionName "C function name"; ChannelName "Channel (pin) name"
      mask Display: disp('EHOOKS FlexECU\nDevLib Wrapper\nS-Function')
  Gain : Gain  Gain=5/1023  OutDataTypeStr=Inherit: Same as input
  status : Outport
  uRaw : Outport  Port=2
  wires:
  Gain/1 -> uRaw/1
  Data Type Conversion2/1 -> Gain/1
  Data Type Conversion3/1 -> status/1
  FlexECU_DevLib_FcnAPI_Wrapper_SFcn/1 -> Data Type Conversion3/1
  FlexECU_DevLib_FcnAPI_Wrapper_SFcn/2 -> Data Type Conversion2/1

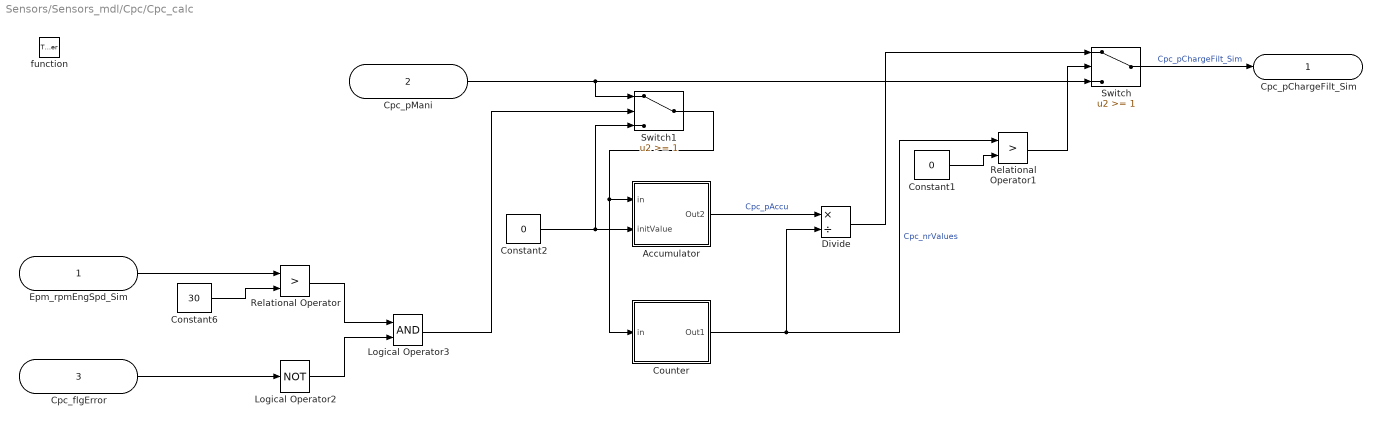
== system Sensors/Sensors_mdl/Cpc/Cpc_calc ==
  Epm_rpmEngSpd_Sim : Inport
  Cpc_pMani : Inport  Port=2
  Cpc_flgError : Inport  Port=3
  function : TriggerPort  TriggerType=function-call  VariantControl=(inherit)
  Accumulator : Subsystem
      mask help: Accumulator
      mask Display: image(imread('Accumulator.jpg'))
  Constant1 : Constant  Value=0  OutDataTypeStr=single
  Constant2 : Constant  Value=0  OutDataTypeStr=single
  Constant6 : Constant  Value=30  OutDataTypeStr=single
  Counter : Subsystem
      mask help: Counter
      mask Display: image(imread('Counter.jpg'))
  Divide : Product  Inputs=*/  OutDataTypeStr=single
  Logical Operator2 : Logic  Operator=NOT  AllPortsSameDT=off  OutDataTypeStr=boolean
  Logical Operator3 : Logic  AllPortsSameDT=off  OutDataTypeStr=boolean
  Relational Operator : RelationalOperator  Operator=>  OutDataTypeStr=boolean  RndMeth=Nearest
  Relational Operator1 : RelationalOperator  Operator=>  OutDataTypeStr=boolean  RndMeth=Nearest
  Switch : Switch  Threshold=1
  Switch1 : Switch  Threshold=1
  Cpc_pChargeFilt_Sim : Outport
  wires:
  Cpc_flgError/1 -> Logical Operator2/1
  Cpc_pMani/1 -> Switch1/1, Switch/3
  Logical Operator2/1 -> Logical Operator3/2
  Relational Operator/1 -> Logical Operator3/1
  Epm_rpmEngSpd_Sim/1 -> Relational Operator/1
  Constant6/1 -> Relational Operator/2
  Counter/1(Out1) -> Divide/2, Relational Operator1/1  "Cpc_nrValues"
  Constant1/1 -> Relational Operator1/2
  Relational Operator1/1 -> Switch/2
  Constant2/1 -> Accumulator/2(initValue), Switch1/3
  Accumulator/1(Out2) -> Divide/1  "Cpc_pAccu"
  Switch/1 -> Cpc_pChargeFilt_Sim/1  "Cpc_pChargeFilt_Sim"
  Divide/1 -> Switch/1
  Logical Operator3/1 -> Switch1/2
  Switch1/1 -> Accumulator/1(in), Counter/1(in)

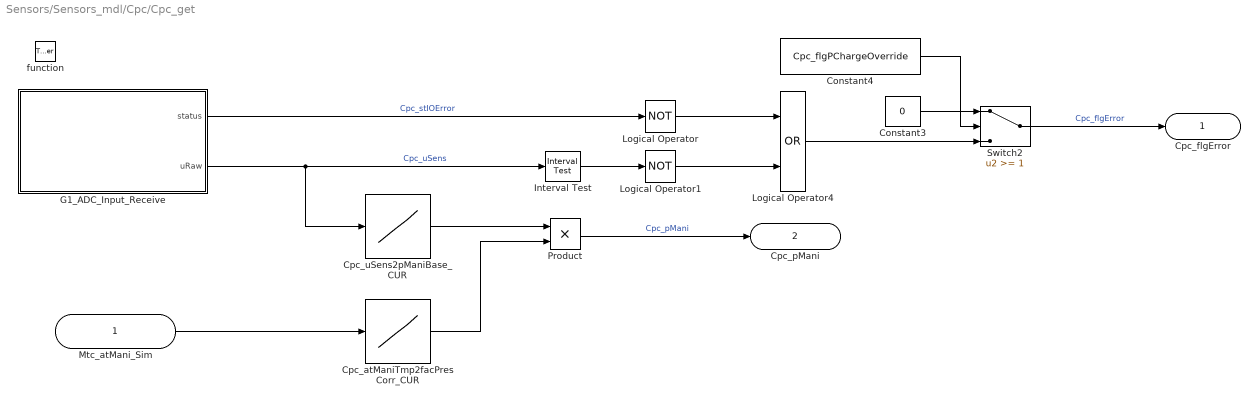
== system Sensors/Sensors_mdl/Cpc/Cpc_get ==
  Mtc_atMani_Sim : Inport
  function : TriggerPort  TriggerType=function-call  VariantControl=(inherit)
  Constant3 : Constant  Value=0  OutDataTypeStr=boolean
  Constant4 : Constant  Value=Cpc_flgPChargeOverride
  Cpc_atManiTmp2facPresCorr_CUR : Lookup_n-D  NumberOfTableDimensions=1  BreakpointsForDimension1=[1:3]  BreakpointsForDimension1DataTypeStr=Inherit: Inherit from 'Breakpoint data'  Table=[6 4 9]  TableDataTypeStr=Inherit: Inherit from 'Table data'  ExtrapMethod=Clip  OutDataTypeStr=Inherit: Inherit from 'Table data'  InputSameDT=on
  Cpc_uSens2pManiBase_CUR : Lookup_n-D  NumberOfTableDimensions=1  BreakpointsForDimension1=[1:3]  BreakpointsForDimension1DataTypeStr=Inherit: Inherit from 'Breakpoint data'  Table=[1 2 5]  TableDataTypeStr=Inherit: Inherit from 'Table data'  ExtrapMethod=Clip  OutDataTypeStr=Inherit: Inherit from 'Table data'  InputSameDT=on
  G1_ADC_Input_Receive : Subsystem  mask{ChannelName=I_A_AN05}
      mask prompts: ChannelName "Channel name"
      mask init:
      | ehooks_medc17flex_devlib_io_block('mask_init');
      settings: AttributesFormatString=Channel name: '%<ChannelName>'
      mask TypeOptions ChannelName: <empty> | I_A_AN01 | I_A_AN02 | I_A_AN03 | I_A_AN05 | I_A_AN06 | I_A_AN07 | I_A_AN08 | I_A_AN10 | I_A_AN11 | I_A_AN12 | I_A_AN13 | I_A_AN14 | I_A_AN15 | I_A_AN16 | I_A_AN17 | I_A_AN18 | I_A_AN19 | I_A_AN20 | I_A_AN21 | I_A_AN23 | I_A_AN32 | I_A_AN35 | I_A_AN36 | I_A_AN37 | I_A_AN39 | I_A_AN100 | I_A_AN101 | I_A_AN103 | I_A_AN104 | I_A_AN105 | I_A_AN106
      mask Display: image(imread('Input_Analog.jpg'))
  Interval Test : simulink/Logic and Bit Operations/Interval Test  IntervalClosedRight=on  uplimit=Mpc_uSensMaxValid  IntervalClosedLeft=on  lowlimit=Mpc_uSensMinValid  OutDataTypeStr=boolean
  Logical Operator : Logic  Operator=NOT  AllPortsSameDT=off  OutDataTypeStr=boolean
  Logical Operator1 : Logic  Operator=NOT  AllPortsSameDT=off  OutDataTypeStr=boolean
  Logical Operator4 : Logic  Operator=OR  AllPortsSameDT=off  OutDataTypeStr=boolean
  Product : Product  OutDataTypeStr=Inherit: Same as first input
  Switch2 : Switch  Threshold=1
  Cpc_flgError : Outport
  Cpc_pMani : Outport  Port=2
  wires:
  Cpc_atManiTmp2facPresCorr_CUR/1 -> Product/2
  Cpc_uSens2pManiBase_CUR/1 -> Product/1
  Mtc_atMani_Sim/1 -> Cpc_atManiTmp2facPresCorr_CUR/1
  Product/1 -> Cpc_pMani/1  "Cpc_pMani"
  G1_ADC_Input_Receive/1(status) -> Logical Operator/1  "Cpc_stIOError"
  G1_ADC_Input_Receive/2(uRaw) -> Cpc_uSens2pManiBase_CUR/1, Interval Test/1  "Cpc_uSens"
  Interval Test/1 -> Logical Operator1/1
  Logical Operator/1 -> Logical Operator4/1
  Logical Operator1/1 -> Logical Operator4/2
  Switch2/1 -> Cpc_flgError/1  "Cpc_flgError"
  Logical Operator4/1 -> Switch2/3
  Constant3/1 -> Switch2/1
  Constant4/1 -> Switch2/2

== system Sensors/Sensors_mdl/Ctc/G1_ADC_Input_Receive ==
  Data Type Conversion2 : DataTypeConversion  OutMin=0.0  OutMax=5.0  OutDataTypeStr=single
  Data Type Conversion3 : DataTypeConversion  OutMin=0.0  OutMax=1.0  OutDataTypeStr=boolean
  FlexECU_DevLib_FcnAPI_Wrapper_SFcn : S-Function  FunctionName=ehooks_medc17flex_devlib_basic_io_fcncall  Parameters=NoInputPorts, NoOutputPorts, InputPortDataTypes, OutputPortDataTypes, CFunctionArgTypes, CFunctionName, ChannelName  SFunctionDeploymentMode=off  EnableBusSupport=off  mask{NoInputPorts=0, NoOutputPorts=2, InputPortDataTypes=, OutputPortDataTypes=uint8,int16, CFunctionArgTypes=ret,ref, CFunctionName=DevLib_Adc_Get, ChannelName=I_A_AN10}
      mask prompts: NoInputPorts "Number of input ports"; NoOutputPorts "Number of output ports"; InputPortDataTypes "Input port data types"; OutputPortDataTypes "Output port data types"; CFunctionArgTypes "C function argument types"; CFunctionName "C function name"; ChannelName "Channel (pin) name"
      mask Display: disp('EHOOKS FlexECU\nDevLib Wrapper\nS-Function')
  Gain : Gain  Gain=5/1023  OutDataTypeStr=Inherit: Same as input
  status : Outport
  uRaw : Outport  Port=2
  wires:
  FlexECU_DevLib_FcnAPI_Wrapper_SFcn/2 -> Data Type Conversion2/1
  FlexECU_DevLib_FcnAPI_Wrapper_SFcn/1 -> Data Type Conversion3/1
  Data Type Conversion3/1 -> status/1
  Data Type Conversion2/1 -> Gain/1
  Gain/1 -> uRaw/1

== system Sensors/Sensors_mdl/Egc/G1_ADC_Input_Receive ==
  Data Type Conversion : DataTypeConversion  OutMin=0.0  OutMax=5.0  OutDataTypeStr=single
  Data Type Conversion1 : DataTypeConversion  OutMin=0.0  OutMax=1.0  OutDataTypeStr=boolean
  FlexECU_DevLib_FcnAPI_Wrapper_SFcn : S-Function  FunctionName=ehooks_medc17flex_devlib_basic_io_fcncall  Parameters=NoInputPorts, NoOutputPorts, InputPortDataTypes, OutputPortDataTypes, CFunctionArgTypes, CFunctionName, ChannelName  SFunctionDeploymentMode=off  EnableBusSupport=off  mask{NoInputPorts=0, NoOutputPorts=2, InputPortDataTypes=, OutputPortDataTypes=uint8,int16, CFunctionArgTypes=ret,ref, CFunctionName=DevLib_Adc_Get, ChannelName=I_A_AN08}
      mask prompts: NoInputPorts "Number of input ports"; NoOutputPorts "Number of output ports"; InputPortDataTypes "Input port data types"; OutputPortDataTypes "Output port data types"; CFunctionArgTypes "C function argument types"; CFunctionName "C function name"; ChannelName "Channel (pin) name"
      mask Display: disp('EHOOKS FlexECU\nDevLib Wrapper\nS-Function')
  Gain : Gain  Gain=5/1023  OutDataTypeStr=Inherit: Same as input
  status : Outport
  uRaw : Outport  Port=2
  wires:
  Data Type Conversion1/1 -> status/1
  Data Type Conversion/1 -> Gain/1
  FlexECU_DevLib_FcnAPI_Wrapper_SFcn/2 -> Data Type Conversion/1
  FlexECU_DevLib_FcnAPI_Wrapper_SFcn/1 -> Data Type Conversion1/1
  Gain/1 -> uRaw/1

== system Sensors/Sensors_mdl/Egc/G1_ADC_Input_Receive1 ==
  Data Type Conversion : DataTypeConversion  OutMin=0.0  OutMax=5.0  OutDataTypeStr=single
  Data Type Conversion1 : DataTypeConversion  OutMin=0.0  OutMax=1.0  OutDataTypeStr=boolean
  FlexECU_DevLib_FcnAPI_Wrapper_SFcn : S-Function  FunctionName=ehooks_medc17flex_devlib_basic_io_fcncall  Parameters=NoInputPorts, NoOutputPorts, InputPortDataTypes, OutputPortDataTypes, CFunctionArgTypes, CFunctionName, ChannelName  SFunctionDeploymentMode=off  EnableBusSupport=off  mask{NoInputPorts=0, NoOutputPorts=2, InputPortDataTypes=, OutputPortDataTypes=uint8,int16, CFunctionArgTypes=ret,ref, CFunctionName=DevLib_Adc_Get, ChannelName=I_A_AN13}
      mask prompts: NoInputPorts "Number of input ports"; NoOutputPorts "Number of output ports"; InputPortDataTypes "Input port data types"; OutputPortDataTypes "Output port data types"; CFunctionArgTypes "C function argument types"; CFunctionName "C function name"; ChannelName "Channel (pin) name"
      mask Display: disp('EHOOKS FlexECU\nDevLib Wrapper\nS-Function')
  Gain : Gain  Gain=5/1023  OutDataTypeStr=Inherit: Same as input
  status : Outport
  uRaw : Outport  Port=2
  wires:
  Data Type Conversion1/1 -> status/1
  Data Type Conversion/1 -> Gain/1
  FlexECU_DevLib_FcnAPI_Wrapper_SFcn/2 -> Data Type Conversion/1
  FlexECU_DevLib_FcnAPI_Wrapper_SFcn/1 -> Data Type Conversion1/1
  Gain/1 -> uRaw/1

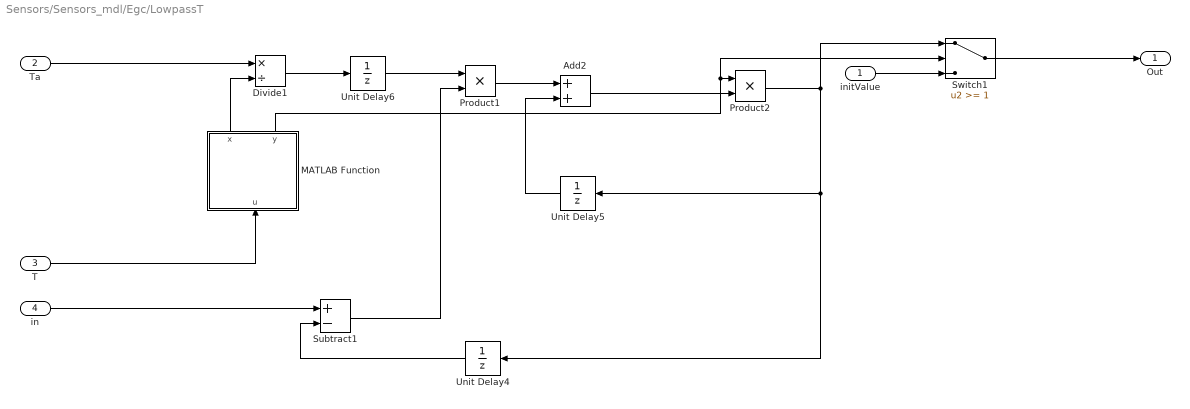
== system Sensors/Sensors_mdl/Egc/LowpassT ==
  initValue : Inport
  Ta : Inport  Port=2
  T : Inport  Port=3
  in : Inport  Port=4
  Add2 : Sum  OutDataTypeStr=Inherit: Same as first input
  Divide1 : Product  Inputs=*/  OutDataTypeStr=Inherit: Same as first input
  MATLAB Function : MATLAB Function  TreatAsAtomicUnit=on
  Product1 : Product  OutDataTypeStr=Inherit: Same as first input
  Product2 : Product  OutDataTypeStr=single
  Subtract1 : Sum  Inputs=+-
  Switch1 : Switch  Threshold=1
  Unit Delay4 : UnitDelay  SampleTime=-1
  Unit Delay5 : UnitDelay  SampleTime=-1
  Unit Delay6 : UnitDelay  SampleTime=-1
  Out : Outport
  wires:
  initValue/1 -> Switch1/3
  Switch1/1 -> Out/1
  MATLAB Function/1(x) -> Divide1/2
  MATLAB Function/2(y) -> Switch1/2, Product2/1
  Ta/1 -> Divide1/1
  T/1 -> MATLAB Function/1(u)
  Divide1/1 -> Unit Delay6/1
  Subtract1/1 -> Product1/2
  Product1/1 -> Add2/1
  Unit Delay5/1 -> Add2/2
  Unit Delay6/1 -> Product1/1
  Unit Delay4/1 -> Subtract1/2
  in/1 -> Subtract1/1
  Product2/1 -> Switch1/1, Unit Delay4/1, Unit Delay5/1
  Add2/1 -> Product2/2

== system Sensors/Sensors_mdl/Egc/LowpassT_Fcn ==
  initValue : Inport
  In : Inport  Port=2
  T : Inport  Port=3
  Discrete Transfer Fcn : DiscreteTransferFcn  Denominator=[Egc_tiTEgasFilt/0.01 1-Egc_tiTEgasFilt/0.01]  OutDataTypeStr=Inherit: Same as input
  MATLAB Function : MATLAB Function  TreatAsAtomicUnit=on
  Product1 : Product  OutDataTypeStr=single
  Switch1 : Switch  Threshold=1
  Out : Outport
  wires:
  MATLAB Function/1(y) -> Switch1/2, Product1/1
  T/1 -> MATLAB Function/1(u)
  initValue/1 -> Switch1/3
  Switch1/1 -> Out/1
  Product1/1 -> Switch1/1
  Discrete Transfer Fcn/1 -> Product1/2
  In/1 -> Discrete Transfer Fcn/1

== system Sensors/Sensors_mdl/Klemme50/G1_Digital_Input_Receive ==
  Data Type Conversion2 : DataTypeConversion  OutMin=0.0  OutMax=1.0  OutDataTypeStr=boolean
  Data Type Conversion3 : DataTypeConversion  OutMin=0.0  OutMax=1.0  OutDataTypeStr=boolean
  FlexECU_DevLib_FcnAPI_Wrapper_SFcn : S-Function  FunctionName=ehooks_medc17flex_devlib_basic_io_fcncall  Parameters=NoInputPorts, NoOutputPorts, InputPortDataTypes, OutputPortDataTypes, CFunctionArgTypes, CFunctionName, ChannelName  SFunctionDeploymentMode=off  EnableBusSupport=off  mask{NoInputPorts=0, NoOutputPorts=2, InputPortDataTypes=, OutputPortDataTypes=uint8,uint8, CFunctionArgTypes=ret,ref, CFunctionName=DevLib_Dio_Get, ChannelName=I_S_DIG17}
      mask prompts: NoInputPorts "Number of input ports"; NoOutputPorts "Number of output ports"; InputPortDataTypes "Input port data types"; OutputPortDataTypes "Output port data types"; CFunctionArgTypes "C function argument types"; CFunctionName "C function name"; ChannelName "Channel (pin) name"
      mask Display: disp('EHOOKS FlexECU\nDevLib Wrapper\nS-Function')
  status : Outport
  stRaw1 : Outport  Port=2
  wires:
  FlexECU_DevLib_FcnAPI_Wrapper_SFcn/2 -> Data Type Conversion2/1
  FlexECU_DevLib_FcnAPI_Wrapper_SFcn/1 -> Data Type Conversion3/1
  Data Type Conversion3/1 -> status/1
  Data Type Conversion2/1 -> stRaw1/1

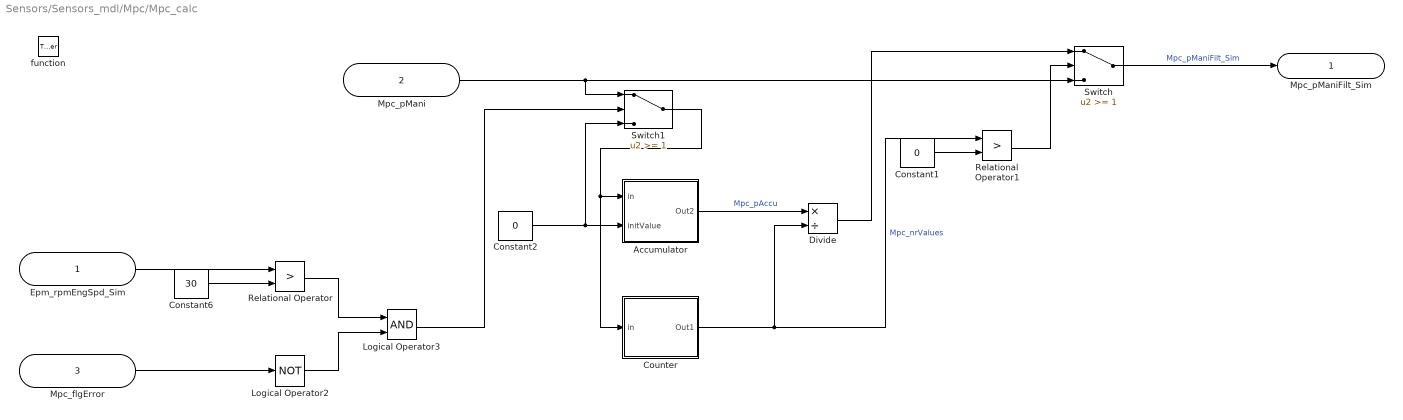
== system Sensors/Sensors_mdl/Mpc/Mpc_calc ==
  Epm_rpmEngSpd_Sim : Inport
  Mpc_pMani : Inport  Port=2
  Mpc_flgError : Inport  Port=3
  function : TriggerPort  TriggerType=function-call  VariantControl=(inherit)
  Accumulator : Subsystem
      mask help: Accumulator
      mask Display: image(imread('Accumulator.jpg'))
  Constant1 : Constant  Value=0  OutDataTypeStr=single
  Constant2 : Constant  Value=0  OutDataTypeStr=single
  Constant6 : Constant  Value=30  OutDataTypeStr=single
  Counter : Subsystem
      mask help: Counter
      mask Display: image(imread('Counter.jpg'))
  Divide : Product  Inputs=*/  OutDataTypeStr=single
  Logical Operator2 : Logic  Operator=NOT  AllPortsSameDT=off  OutDataTypeStr=boolean
  Logical Operator3 : Logic  AllPortsSameDT=off  OutDataTypeStr=boolean
  Relational Operator : RelationalOperator  Operator=>  OutDataTypeStr=boolean  RndMeth=Nearest
  Relational Operator1 : RelationalOperator  Operator=>  OutDataTypeStr=boolean  RndMeth=Nearest
  Switch : Switch  Threshold=1
  Switch1 : Switch  Threshold=1
  Mpc_pManiFilt_Sim : Outport
  wires:
  Switch1/1 -> Counter/1(in), Accumulator/1(in)
  Logical Operator3/1 -> Switch1/2
  Divide/1 -> Switch/1
  Switch/1 -> Mpc_pManiFilt_Sim/1  "Mpc_pManiFilt_Sim"
  Accumulator/1(Out2) -> Divide/1  "Mpc_pAccu"
  Constant2/1 -> Switch1/3, Accumulator/2(initValue)
  Relational Operator1/1 -> Switch/2
  Constant1/1 -> Relational Operator1/2
  Counter/1(Out1) -> Relational Operator1/1, Divide/2  "Mpc_nrValues"
  Constant6/1 -> Relational Operator/2
  Epm_rpmEngSpd_Sim/1 -> Relational Operator/1
  Relational Operator/1 -> Logical Operator3/1
  Logical Operator2/1 -> Logical Operator3/2
  Mpc_pMani/1 -> Switch/3, Switch1/1
  Mpc_flgError/1 -> Logical Operator2/1

== system Sensors/Sensors_mdl/Mpc/Mpc_get ==
  Mtc_atMani_Sim : Inport
  function : TriggerPort  TriggerType=function-call  VariantControl=(inherit)
  G1_ADC_Input_Receive : Subsystem  mask{ChannelName=I_A_AN05}
      mask prompts: ChannelName "Channel name"
      mask init:
      | ehooks_medc17flex_devlib_io_block('mask_init');
      settings: AttributesFormatString=Channel name: '%<ChannelName>'
      mask TypeOptions ChannelName: <empty> | I_A_AN01 | I_A_AN02 | I_A_AN03 | I_A_AN05 | I_A_AN06 | I_A_AN07 | I_A_AN08 | I_A_AN10 | I_A_AN11 | I_A_AN12 | I_A_AN13 | I_A_AN14 | I_A_AN15 | I_A_AN16 | I_A_AN17 | I_A_AN18 | I_A_AN19 | I_A_AN20 | I_A_AN21 | I_A_AN23 | I_A_AN32 | I_A_AN35 | I_A_AN36 | I_A_AN37 | I_A_AN39 | I_A_AN100 | I_A_AN101 | I_A_AN103 | I_A_AN104 | I_A_AN105 | I_A_AN106
      mask Display: image(imread('Input_Analog.jpg'))
  Interval Test : simulink/Logic and Bit Operations/Interval Test  IntervalClosedRight=on  uplimit=Mpc_uSensMaxValid  IntervalClosedLeft=on  lowlimit=Mpc_uSensMinValid  OutDataTypeStr=boolean
  Logical Operator : Logic  Operator=NOT  AllPortsSameDT=off  OutDataTypeStr=boolean
  Logical Operator1 : Logic  Operator=NOT  AllPortsSameDT=off  OutDataTypeStr=boolean
  Logical Operator4 : Logic  Operator=OR  AllPortsSameDT=off  OutDataTypeStr=boolean
  Mpc_atManiTmp2facPresCorr_CUR : Lookup_n-D  NumberOfTableDimensions=1  BreakpointsForDimension1=[1:3]  BreakpointsForDimension1DataTypeStr=Inherit: Inherit from 'Breakpoint data'  Table=[1 3 8]  TableDataTypeStr=Inherit: Inherit from 'Table data'  ExtrapMethod=Clip  OutDataTypeStr=Inherit: Inherit from 'Table data'  InputSameDT=on
  Mpc_uSens2pManiBase_CUR : Lookup_n-D  NumberOfTableDimensions=1  BreakpointsForDimension1=[1:3]  BreakpointsForDimension1DataTypeStr=Inherit: Inherit from 'Breakpoint data'  Table=[1 4 5]  TableDataTypeStr=Inherit: Inherit from 'Table data'  ExtrapMethod=Clip  OutDataTypeStr=Inherit: Inherit from 'Table data'  InputSameDT=on
  Product : Product  OutDataTypeStr=Inherit: Same as first input
  Mpc_flgError : Outport
  Mpc_pMani : Outport  Port=2
  wires:
  Logical Operator4/1 -> Mpc_flgError/1  "Mpc_flgError"
  Logical Operator1/1 -> Logical Operator4/2
  Logical Operator/1 -> Logical Operator4/1
  Interval Test/1 -> Logical Operator1/1
  G1_ADC_Input_Receive/2(uRaw) -> Mpc_uSens2pManiBase_CUR/1, Interval Test/1  "Mpc_uSens"
  G1_ADC_Input_Receive/1(status) -> Logical Operator/1  "Mpc_stIOError"
  Product/1 -> Mpc_pMani/1  "Mpc_pMani"
  Mtc_atMani_Sim/1 -> Mpc_atManiTmp2facPresCorr_CUR/1
  Mpc_uSens2pManiBase_CUR/1 -> Product/1
  Mpc_atManiTmp2facPresCorr_CUR/1 -> Product/2

== system Sensors/Sensors_mdl/Mtc/G1_ADC_Input_Receive ==
  Data Type Conversion2 : DataTypeConversion  OutMin=0.0  OutMax=5.0  OutDataTypeStr=single
  Data Type Conversion3 : DataTypeConversion  OutMin=0.0  OutMax=1.0  OutDataTypeStr=boolean
  FlexECU_DevLib_FcnAPI_Wrapper_SFcn : S-Function  FunctionName=ehooks_medc17flex_devlib_basic_io_fcncall  Parameters=NoInputPorts, NoOutputPorts, InputPortDataTypes, OutputPortDataTypes, CFunctionArgTypes, CFunctionName, ChannelName  SFunctionDeploymentMode=off  EnableBusSupport=off  mask{NoInputPorts=0, NoOutputPorts=2, InputPortDataTypes=, OutputPortDataTypes=uint8,int16, CFunctionArgTypes=ret,ref, CFunctionName=DevLib_Adc_Get, ChannelName=I_A_AN14}
      mask prompts: NoInputPorts "Number of input ports"; NoOutputPorts "Number of output ports"; InputPortDataTypes "Input port data types"; OutputPortDataTypes "Output port data types"; CFunctionArgTypes "C function argument types"; CFunctionName "C function name"; ChannelName "Channel (pin) name"
      mask Display: disp('EHOOKS FlexECU\nDevLib Wrapper\nS-Function')
  Gain : Gain  Gain=5/1023  OutDataTypeStr=Inherit: Same as input
  status : Outport
  uRaw : Outport  Port=2
  wires:
  FlexECU_DevLib_FcnAPI_Wrapper_SFcn/1 -> Data Type Conversion3/1
  FlexECU_DevLib_FcnAPI_Wrapper_SFcn/2 -> Data Type Conversion2/1
  Gain/1 -> uRaw/1
  Data Type Conversion3/1 -> status/1
  Data Type Conversion2/1 -> Gain/1
